simulink model "cftest"  (R2019b)
settings: Solver=FixedStepAuto  StartTime=0.0  StopTime=10.0  FixedStep=0.1  RelTol=1e-3
InitFcn:
  | cf_init
libraries: simulink x3
settings Model: Creator=paul  LastModifiedBy=paul

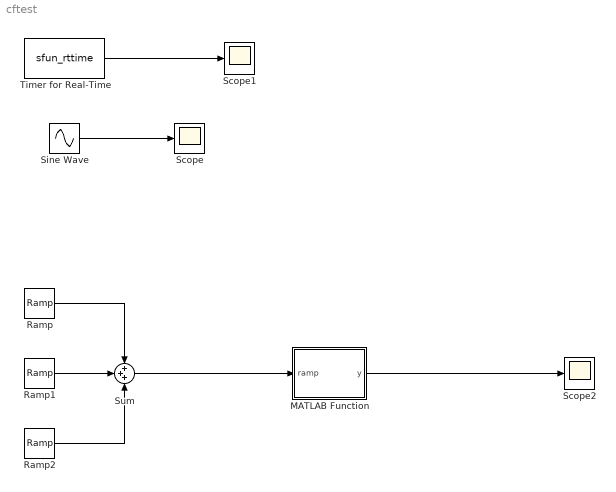
== system cftest ==
  MATLAB Function : MATLAB Function  TreatAsAtomicUnit=on
  Ramp : simulink/Sources/Ramp  slope=3000  start=1  InitialOutput=0
  Ramp1 : simulink/Sources/Ramp  slope=-6000  start=4  InitialOutput=0
  Ramp2 : simulink/Sources/Ramp  slope=3000  start=7  InitialOutput=0
  Scope : Scope
  Scope1 : Scope
  Scope2 : Scope
  Sine Wave : Sin  SampleTime=0
  Sum : Sum  Inputs=+++
  Timer for Real-Time : S-Function  FunctionName=sfun_rttime  Parameters=1  SFunctionDeploymentMode=off  EnableBusSupport=off
  wires:
  Sine Wave/1 -> Scope/1
  Timer for Real-Time/1 -> Scope1/1
  Ramp1/1 -> Sum/2
  Ramp/1 -> Sum/1
  Ramp2/1 -> Sum/3
  Sum/1 -> MATLAB Function/1(ramp)
  MATLAB Function/1(y) -> Scope2/1

== matlab function cftest/MATLAB Function ==
  data: ramp input; y output; a parameter
function y = fcn(ramp,a)

coder.extrinsic('py.list') 

a.commander.send_setpoint(0,0,0,ramp);

y = ramp;
